simulink model "untitled"  (R2019b)
settings: Solver=VariableStepAuto  StartTime=0.0  StopTime=10.0  RelTol=1e-3
settings Model: Creator=edmon  LastModifiedBy=edmon

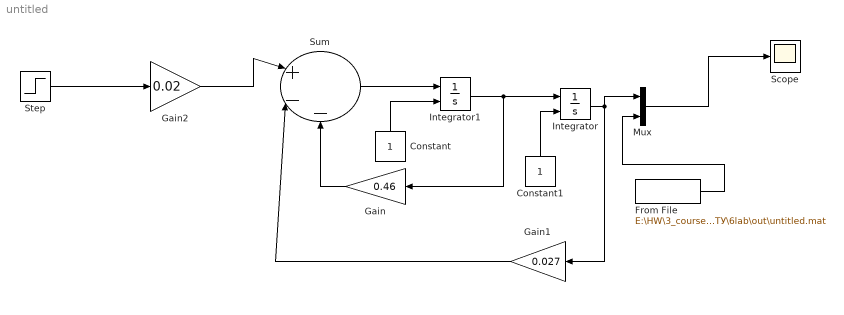
== system untitled ==
  Constant : Constant
  Constant1 : Constant
  From File : FromFile  FileName=E:\HW\3_course\ОТУ\6lab\out\untitled.mat  SampleTime=0
  Gain : Gain  Gain=0.46
  Gain1 : Gain  Gain=0.027
  Gain2 : Gain  Gain=0.02
  Integrator : Integrator  ExternalReset=level hold
  Integrator1 : Integrator  ExternalReset=level hold
  Mux : Mux  Inputs=2
  Scope : Scope
  Step : Step  SampleTime=0
  Sum : Sum  Inputs=|+--
  wires:
  Integrator1/1 -> Integrator/1, Gain/1
  Gain1/1 -> Sum/2
  Gain/1 -> Sum/3
  Integrator/1 -> Mux/1, Gain1/1
  Gain2/1 -> Sum/1
  Step/1 -> Gain2/1
  Constant/1 -> Integrator1/2
  Sum/1 -> Integrator1/1
  Constant1/1 -> Integrator/2
  Mux/1 -> Scope/1
  From File/1 -> Mux/2
